simulink model "AFM_SS_linearFDBK_obs"  (R2016b)
settings: Solver=VariableStepDiscrete  StartTime=0.0  StopTime=trun  FixedStep=Ts  EnableMultiTasking=on
undefined symbols (not defined in the file): absorbDelay, C_delay, H, K, Ki, L, Nbar, Nd_out, Ns, PLANT, sys_obs, Ts, umax, x0_int, X0_obs, x0_obs
libraries: powerlib_meascontrol x1, cstblocks x1
settings Model: Creator=arnold  LastModifiedBy=arnold
settings DataIOCC: SaveFormat=Structure  SaveOutput=off  SaveState=on  InspectSignalLogs=on  TimeSaveName=tout_ptos
settings OptimizationCC: LifeSpan=inf
settings DebuggingCC: SolverPrmCheckMsg=warning  SFUnexpectedBacktrackingDiag=warning  SFNoUnconditionalDefaultTransitionDiag=warning  SFExecutionAtInitializationDiag=none
settings HardwareCC: ProdBitPerPointer=32  ProdBitPerSizeT=32  ProdBitPerPtrDiffT=32  ProdLargestAtomicFloat=None  ProdIntDivRoundTo=Undefined  ProdEndianess=Unspecified  ProdWordSize=32  ProdHWDeviceType=32-bit Generic
settings ModelReferenceCC: PropagateSignalLabelsOutOfModel=off
settings GRTTargetCC: TargetLangStandard=C89/C90 (ANSI)  GeneratePreprocessorConditionals=Disable all
settings ConfigComp: CovMetricSettings=dw  CovHtmlReporting=on  CovSaveCumulativeToWorkspaceVar=on  CovSaveSingleToWorkspaceVar=on  CovExternalEMLEnable=off  CovSFcnEnable=off

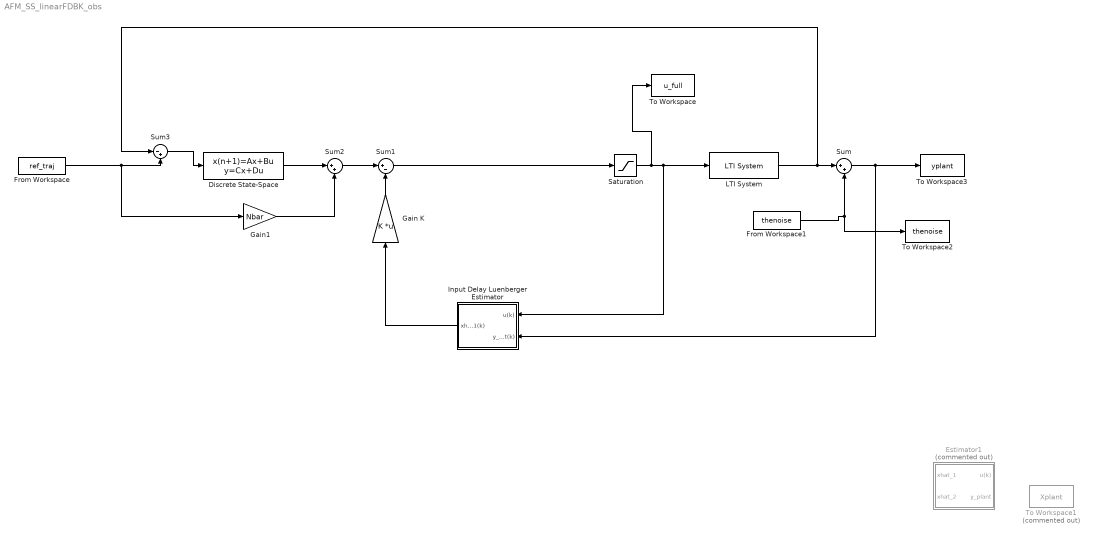
== system AFM_SS_linearFDBK_obs ==
  Discrete State-Space : DiscreteStateSpace  B=Ki  D=0  X0=x0_int  SampleTime=Ts
  Estimator1 : Subsystem  Commented=on
  From Workspace : FromWorkspace  VariableName=ref_traj  SampleTime=Ts
  From Workspace1 : FromWorkspace  VariableName=thenoise  SampleTime=Ts
  Gain K : Gain  Gain=K  Multiplication=Matrix(K*u)
  Gain1 : Gain  Gain=Nbar
  Input Delay Luenberger Estimator : Subsystem  AncestorBlock=customLibFcns/Input Delay Luenberger Estimator
  LTI System : cstblocks/LTI System  sys=absorbDelay(PLANT)  IC=x0_full
  Saturation : Saturate  UpperLimit=umax  LowerLimit=-umax
  Sum : Sum  Inputs=|++
  Sum1 : Sum  Inputs=|+-
  Sum2 : Sum  Inputs=|++
  Sum3 : Sum  Inputs=|-+
  To Workspace : ToWorkspace  VariableName=u_full  SaveFormat=Timeseries  SampleTime=-1
      settings: Save2DSignal=2-D array (concatenate along first dimension)
  To Workspace1 : ToWorkspace  Commented=on  VariableName=Xplant  SaveFormat=Timeseries  SampleTime=-1
      settings: Save2DSignal=2-D array (concatenate along first dimension)
  To Workspace2 : ToWorkspace  VariableName=thenoise  SaveFormat=Timeseries  SampleTime=-1
      settings: Save2DSignal=2-D array (concatenate along first dimension)
  To Workspace3 : ToWorkspace  VariableName=yplant  SaveFormat=Timeseries  SampleTime=-1
      settings: Save2DSignal=2-D array (concatenate along first dimension)
  wires:
  LTI System/1 -> Sum/1, Sum3/1
  Gain K/1 -> Sum1/2
  Input Delay Luenberger Estimator/1(xhat_1(k)) -> Gain K/1
  From Workspace/1 -> Gain1/1, Sum3/2
  Sum3/1 -> Discrete State-Space/1
  Gain1/1 -> Sum2/2
  Sum/1 -> Input Delay Luenberger Estimator/2(y_plant(k)), To Workspace3/1
  From Workspace1/1 -> To Workspace2/1, Sum/2
  Saturation/1 -> To Workspace/1, Input Delay Luenberger Estimator/1(u(k)), LTI System/1
  Sum1/1 -> Saturation/1
  Discrete State-Space/1 -> Sum2/1
  Sum2/1 -> Sum1/1

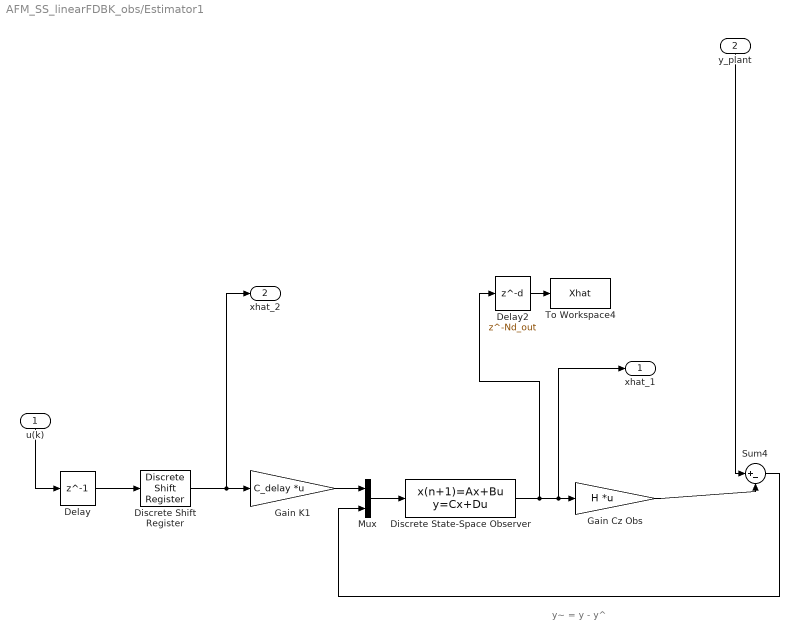
== system AFM_SS_linearFDBK_obs/Estimator1 ==
  note: y~ = y - y^
  u(k) : Inport
  y_plant : Inport  Port=2
  Delay : Delay  DelayLength=1
  Delay2 : Delay  DelayLength=Nd_out
  Discrete Shift Register : powerlib_meascontrol/Additional Components/Discrete Shift Register  NSamples=Nd  InitialValue=0  Ts=Ts
  Discrete State-Space Observer : DiscreteStateSpace  A=sys_obs.a  B=[sys_obs.b, L]  C=eye(Ns)  D=zeros(Ns,2)  X0=X0_obs  SampleTime=Ts
  Gain Cz Obs : Gain  Gain=H  Multiplication=Matrix(K*u)
  Gain K1 : Gain  Gain=C_delay  Multiplication=Matrix(K*u)
  Mux : Mux  Inputs=2
  Sum4 : Sum  Inputs=|+-
  To Workspace4 : ToWorkspace  VariableName=Xhat  SaveFormat=Timeseries  SampleTime=-1
      settings: Save2DSignal=2-D array (concatenate along first dimension)
  xhat_1 : Outport
  xhat_2 : Outport  Port=2
  wires:
  Mux/1 -> Discrete State-Space Observer/1
  Sum4/1 -> Mux/2
  Discrete State-Space Observer/1 -> Delay2/1, Gain Cz Obs/1, xhat_1/1
  y_plant/1 -> Sum4/1
  Gain Cz Obs/1 -> Sum4/2
  Delay2/1 -> To Workspace4/1
  Discrete Shift Register/1 -> xhat_2/1, Gain K1/1
  Delay/1 -> Discrete Shift Register/1
  Gain K1/1 -> Mux/1
  u(k)/1 -> Delay/1

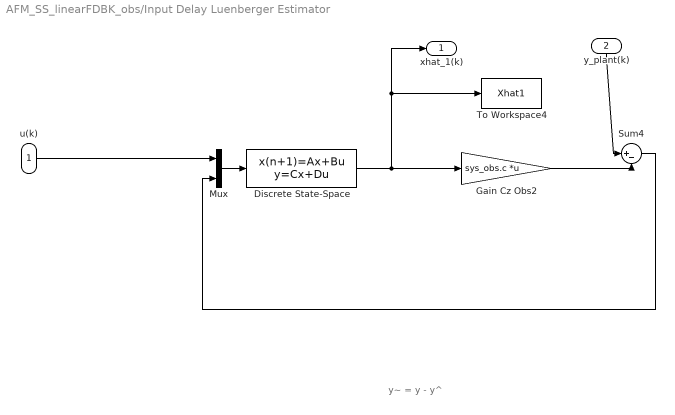
== system AFM_SS_linearFDBK_obs/Input Delay Luenberger Estimator ==
  note: y~ = y - y^
  u(k) : Inport
  y_plant(k) : Inport  Port=2
  Discrete State-Space : DiscreteStateSpace  A=sys_obs.a  B=[sys_obs.b, L]  C=eye(length(sys_obs.b))  D=zeros(length(sys_obs.b), 2)  X0=x0_obs  SampleTime=Ts
  Gain Cz Obs2 : Gain  Gain=sys_obs.c  Multiplication=Matrix(K*u)
  Mux : Mux  Inputs=2
  Sum4 : Sum  Inputs=|+-
  To Workspace4 : ToWorkspace  VariableName=Xhat1  SaveFormat=Timeseries  SampleTime=-1
      settings: Save2DSignal=2-D array (concatenate along first dimension)
  xhat_1(k) : Outport
  wires:
  Sum4/1 -> Mux/2
  u(k)/1 -> Mux/1
  Mux/1 -> Discrete State-Space/1
  Discrete State-Space/1 -> Gain Cz Obs2/1, To Workspace4/1, xhat_1(k)/1
  Gain Cz Obs2/1 -> Sum4/2
  y_plant(k)/1 -> Sum4/1
